simulink model "reaktorChemiczny_20221205_2206"  (R2021b)
settings: Solver=VariableStepAuto  StartTime=0.0  StopTime=10  RelTol=1e-3
model mask{alfa=alfa, ar=ar, cpc=cpc, cpr=cpr, E1=E1, E3=E3, E2=E2, h1=h1, h2=h2, h3=h3, k01=k01, k02=k02, k03=k03, mc=mc, pr=pr, qr=qr, tri=tri, vr=vr}
model workspace (MAT data in the model file):
  E1 = 9800
  E2 = 9800
  E3 = 8600
  Sig = Simulink.Signal
  Sig.DataType = 'auto'
  Sig.Dimensions = -1
  Sig.DimensionsMode = 'auto'
  Sig.Complexity = 'auto'
  Sig.SampleTime = -1
  Sig.SamplingMode = 'auto'
  Sig1 = Simulink.Signal
  Sig1.DataType = 'auto'
  Sig1.Dimensions = -1
  Sig1.DimensionsMode = 'auto'
  Sig1.Complexity = 'auto'
  Sig1.SampleTime = -1
  Sig1.SamplingMode = 'auto'
  alfa = 300
  ar = 0.1
  cpc = 2
  cpr = 3
  h1 = -4200
  h2 = 11000
  h3 = 42000
  k01 = 350000000
  k02 = 350000000
  k03 = 2500000
  mc = 5
  pr = 900
  qr = 0.001
  tri = 393
  vr = 1
settings Model: ParameterArgumentNames=E1,E2,E3,alfa,ar,cpc,cpr,h1,h2,h3,k01,k02,k03,mc,pr,qr,tri,vr  Creator=apple  LastModifiedBy=Black

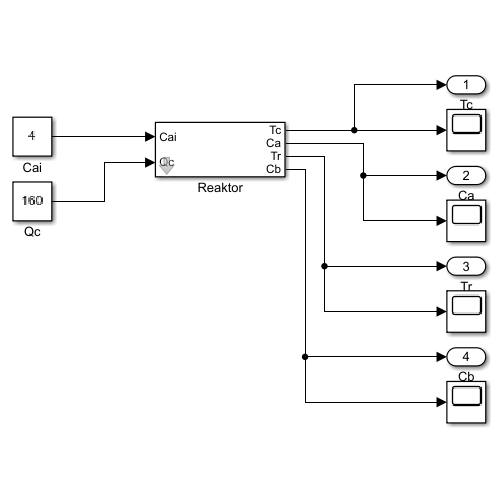
[thumbnail: Simulink's stored preview of the top-level diagram]
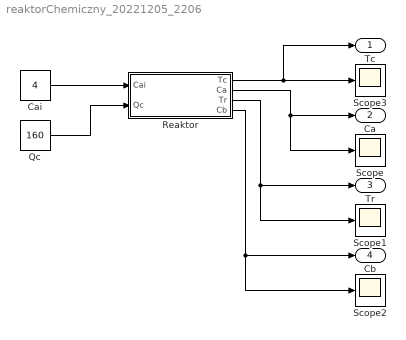
== system reaktorChemiczny_20221205_2206 ==
  Cai : Constant  Value=4
  Qc : Constant  Value=160
  Reaktor : Subsystem  mask{tr0=393, tc0=392, Ca0=5, Cb0=0}
  Scope{,1..3} (4 alike) : Scope
  Tc : Outport
  Ca : Outport  Port=2
  Tr : Outport  Port=3
  Cb : Outport  Port=4
  wires:
  Reaktor/1(Tc) -> Tc/1, Scope3/1
  Reaktor/2(Ca) -> Ca/1, Scope/1
  Reaktor/3(Tr) -> Scope1/1, Tr/1
  Reaktor/4(Cb) -> Scope2/1, Cb/1
  Cai/1 -> Reaktor/1(Cai)
  Qc/1 -> Reaktor/2(Qc)

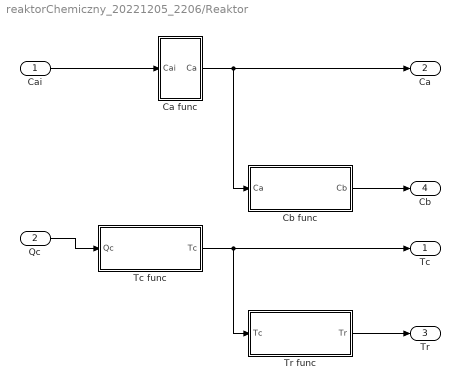
== system reaktorChemiczny_20221205_2206/Reaktor ==
  Cai : Inport  OutMin=0
  Qc : Inport  Port=2  OutMin=0
  Ca func : Subsystem
  Cb func : Subsystem
  Tc func : Subsystem
  Tr func : Subsystem
  Tc : Outport
  Ca : Outport  Port=2
  Tr : Outport  Port=3
  Cb : Outport  Port=4
  wires:
  Tc func/1(Tc) -> Tc/1, Tr func/1(Tc)
  Ca func/1(Ca) -> Cb func/1(Ca), Ca/1
  Cb func/1(Cb) -> Cb/1
  Tr func/1(Tr) -> Tr/1
  Cai/1 -> Ca func/1(Cai)
  Qc/1 -> Tc func/1(Qc)

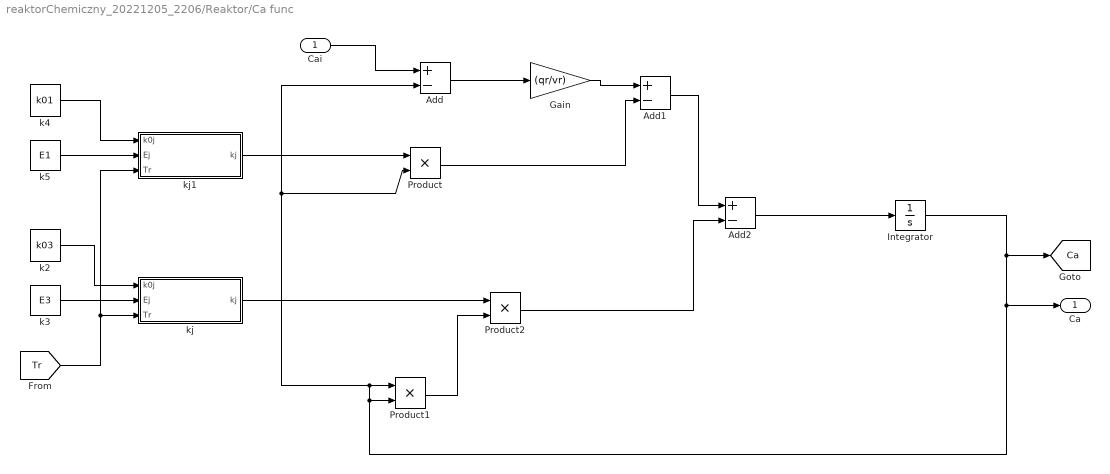
== system reaktorChemiczny_20221205_2206/Reaktor/Ca func ==
  Cai : Inport
  Add : Sum  Inputs=+-
  Add1 : Sum  Inputs=+-
  Add2 : Sum  Inputs=+-
  Gain : Gain  Gain=(qr/vr)
  Integrator : Integrator  InitialCondition=Ca0
  Product : Product
  Product1 : Product
  Product2 : Product
  k2 : Constant  Value=k03
  k3 : Constant  Value=E3
  k4 : Constant  Value=k01
  k5 : Constant  Value=E1
  kj : Subsystem
  kj1 : Subsystem
  Ca : Outport
  tag scope: Ca=global
  wires:
  kj1/1(kj) -> Product/1
  Gain/1 -> Add1/1
  Product1/1 -> Product2/2
  Cai/1 -> Add/1
  Integrator/1 -> [Ca], Ca/1, Product1/1, Add/2, Product/2, Product1/2
  kj/1(kj) -> Product2/1
  Add1/1 -> Add2/1
  Add2/1 -> Integrator/1
  Product2/1 -> Add2/2
  Add/1 -> Gain/1
  Product/1 -> Add1/2
  k3/1 -> kj/2(Ej)
  k2/1 -> kj/1(k0j)
  k5/1 -> kj1/2(Ej)
  k4/1 -> kj1/1(k0j)
  [Tr] -> kj1/3(Tr), kj/3(Tr)

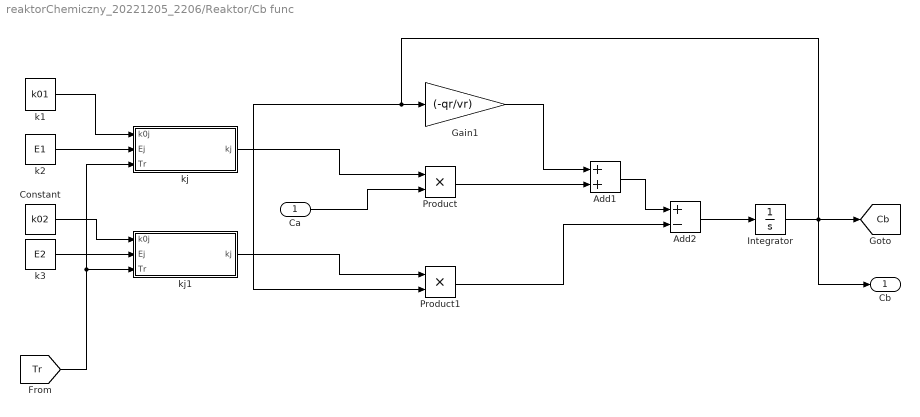
== system reaktorChemiczny_20221205_2206/Reaktor/Cb func ==
  Ca : Inport
  Add1 : Sum
  Add2 : Sum  Inputs=+-
  Constant : Constant  Value=k02
  Gain1 : Gain  Gain=(-qr/vr)
  Integrator : Integrator  InitialCondition=Cb0
  Product : Product
  Product1 : Product
  k1 : Constant  Value=k01
  k2 : Constant  Value=E1
  k3 : Constant  Value=E2
  kj : Subsystem
  kj1 : Subsystem
  Cb : Outport
  tag scope: Cb=global
  wires:
  Add2/1 -> Integrator/1
  Gain1/1 -> Add1/1
  Ca/1 -> Product/2
  Product/1 -> Add1/2
  Integrator/1 -> Product1/2, Gain1/1, [Cb], Cb/1
  Add1/1 -> Add2/1
  Product1/1 -> Add2/2
  k1/1 -> kj/1(k0j)
  Constant/1 -> kj1/1(k0j)
  k2/1 -> kj/2(Ej)
  k3/1 -> kj1/2(Ej)
  [Tr] -> kj1/3(Tr), kj/3(Tr)
  kj1/1(kj) -> Product1/1
  kj/1(kj) -> Product/1

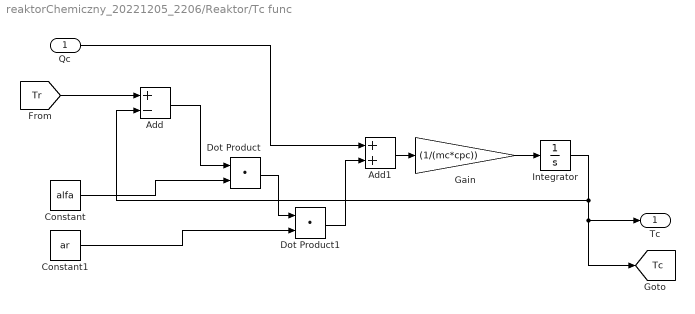
== system reaktorChemiczny_20221205_2206/Reaktor/Tc func ==
  Qc : Inport
  Add : Sum  Inputs=+-
  Add1 : Sum
  Constant : Constant  Value=alfa
  Constant1 : Constant  Value=ar
  Dot Product : DotProduct  InputSameDT=on  OutDataTypeStr=Inherit: Inherit via internal rule
  Dot Product1 : DotProduct  InputSameDT=on  OutDataTypeStr=Inherit: Inherit via internal rule
  Gain : Gain  Gain=(1/(mc*cpc))
  Integrator : Integrator  InitialCondition=tc0
  Tc : Outport
  tag scope: Tc=global
  wires:
  Integrator/1 -> [Tc], Tc/1, Add/2
  Add/1 -> Dot Product/1
  Constant/1 -> Dot Product/2
  Dot Product/1 -> Dot Product1/1
  Constant1/1 -> Dot Product1/2
  Qc/1 -> Add1/1
  Dot Product1/1 -> Add1/2
  Add1/1 -> Gain/1
  Gain/1 -> Integrator/1
  [Tr] -> Add/1

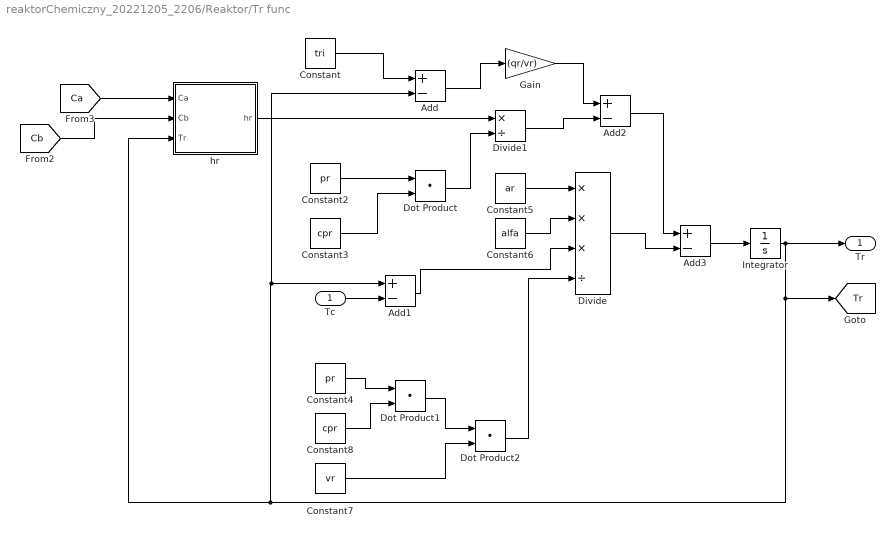
== system reaktorChemiczny_20221205_2206/Reaktor/Tr func ==
  Tc : Inport
  Add{,1..3} (4 alike) : Sum  Inputs=+-
  Constant : Constant  Value=tri
  Constant2 : Constant  Value=pr
  Constant3 : Constant  Value=cpr
  Constant4 : Constant  Value=pr
  Constant5 : Constant  Value=ar
  Constant6 : Constant  Value=alfa
  Constant7 : Constant  Value=vr
  Constant8 : Constant  Value=cpr
  Divide : Product  Inputs=***/
  Divide1 : Product  Inputs=*/
  Dot Product : DotProduct  InputSameDT=on  OutDataTypeStr=Inherit: Inherit via internal rule
  Dot Product1 : DotProduct  InputSameDT=on  OutDataTypeStr=Inherit: Inherit via internal rule
  Dot Product2 : DotProduct  InputSameDT=on  OutDataTypeStr=Inherit: Inherit via internal rule
  Gain : Gain  Gain=(qr/vr)
  Integrator : Integrator  InitialCondition=tr0
  hr : Subsystem
  Tr : Outport
  tag scope: Tr=global
  wires:
  Integrator/1 -> [Tr], Add/2, Add1/1, hr/3(Tr), Tr/1
  Constant/1 -> Add/1
  Constant2/1 -> Dot Product/1
  Constant3/1 -> Dot Product/2
  Dot Product/1 -> Divide1/2
  Divide1/1 -> Add2/2
  Constant5/1 -> Divide/1
  Constant6/1 -> Divide/2
  Add1/1 -> Divide/3
  Constant7/1 -> Dot Product2/2
  Constant4/1 -> Dot Product1/1
  Constant8/1 -> Dot Product1/2
  Dot Product1/1 -> Dot Product2/1
  Dot Product2/1 -> Divide/4
  Tc/1 -> Add1/2
  Divide/1 -> Add3/2
  Add2/1 -> Add3/1
  Add3/1 -> Integrator/1
  Add/1 -> Gain/1
  [Cb] -> hr/2(Cb)
  [Ca] -> hr/1(Ca)
  Gain/1 -> Add2/1
  hr/1(hr) -> Divide1/1

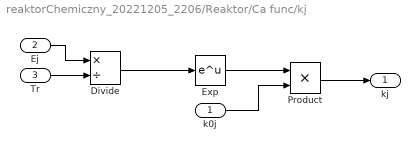
== system reaktorChemiczny_20221205_2206/Reaktor/Ca func/kj ==
  k0j : Inport
  Ej : Inport  Port=2
  Tr : Inport  Port=3
  Divide : Product  Inputs=*/
  Exp : Math  SignedPower=on  SaturateOnIntegerOverflow=on
  Product : Product
  kj : Outport
  wires:
  Product/1 -> kj/1
  Exp/1 -> Product/1
  k0j/1 -> Product/2
  Ej/1 -> Divide/1
  Divide/1 -> Exp/1
  Tr/1 -> Divide/2

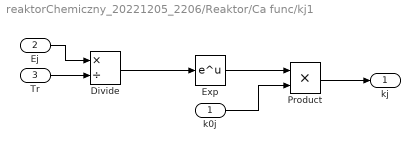
== system reaktorChemiczny_20221205_2206/Reaktor/Ca func/kj1 ==
  k0j : Inport
  Ej : Inport  Port=2
  Tr : Inport  Port=3
  Divide : Product  Inputs=*/
  Exp : Math  SignedPower=on  SaturateOnIntegerOverflow=on
  Product : Product
  kj : Outport
  wires:
  Product/1 -> kj/1
  Exp/1 -> Product/1
  k0j/1 -> Product/2
  Ej/1 -> Divide/1
  Divide/1 -> Exp/1
  Tr/1 -> Divide/2

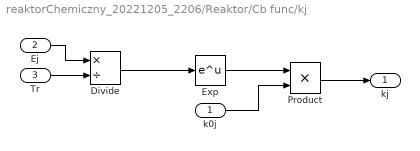
== system reaktorChemiczny_20221205_2206/Reaktor/Cb func/kj ==
  k0j : Inport
  Ej : Inport  Port=2
  Tr : Inport  Port=3
  Divide : Product  Inputs=*/
  Exp : Math  SignedPower=on  SaturateOnIntegerOverflow=on
  Product : Product
  kj : Outport
  wires:
  Product/1 -> kj/1
  Exp/1 -> Product/1
  k0j/1 -> Product/2
  Ej/1 -> Divide/1
  Divide/1 -> Exp/1
  Tr/1 -> Divide/2

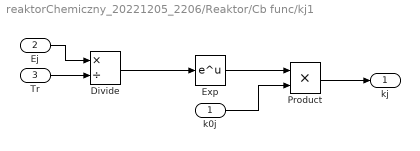
== system reaktorChemiczny_20221205_2206/Reaktor/Cb func/kj1 ==
  k0j : Inport
  Ej : Inport  Port=2
  Tr : Inport  Port=3
  Divide : Product  Inputs=*/
  Exp : Math  SignedPower=on  SaturateOnIntegerOverflow=on
  Product : Product
  kj : Outport
  wires:
  Product/1 -> kj/1
  Exp/1 -> Product/1
  k0j/1 -> Product/2
  Ej/1 -> Divide/1
  Divide/1 -> Exp/1
  Tr/1 -> Divide/2

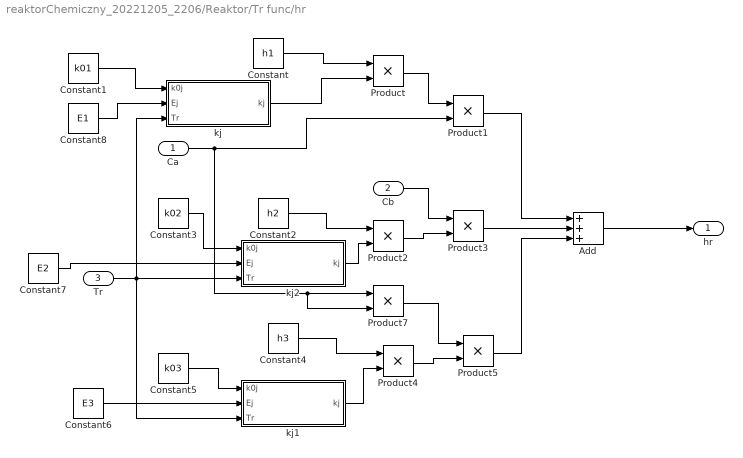
== system reaktorChemiczny_20221205_2206/Reaktor/Tr func/hr ==
  Ca : Inport
  Cb : Inport  Port=2
  Tr : Inport  Port=3
  Add : Sum  Inputs=+++
  Constant : Constant  Value=h1
  Constant1 : Constant  Value=k01
  Constant2 : Constant  Value=h2
  Constant3 : Constant  Value=k02
  Constant4 : Constant  Value=h3
  Constant5 : Constant  Value=k03
  Constant6 : Constant  Value=E3
  Constant7 : Constant  Value=E2
  Constant8 : Constant  Value=E1
  Product{,1..5,7} (7 alike) : Product
  kj : Subsystem
  kj1 : Subsystem
  kj2 : Subsystem
  hr : Outport
  wires:
  Constant/1 -> Product/1
  Product/1 -> Product1/1
  Ca/1 -> Product1/2, Product7/2, Product7/1
  Constant2/1 -> Product2/1
  Product2/1 -> Product3/2
  Cb/1 -> Product3/1
  Product4/1 -> Product5/2
  Constant4/1 -> Product4/1
  Product7/1 -> Product5/1
  Product5/1 -> Add/3
  Product3/1 -> Add/2
  Product1/1 -> Add/1
  Add/1 -> hr/1
  kj/1(kj) -> Product/2
  Constant1/1 -> kj/1(k0j)
  kj1/1(kj) -> Product4/2
  Constant5/1 -> kj1/1(k0j)
  kj2/1(kj) -> Product2/2
  Constant3/1 -> kj2/1(k0j)
  Tr/1 -> kj2/3(Tr), kj/3(Tr), kj1/3(Tr)
  Constant6/1 -> kj1/2(Ej)
  Constant7/1 -> kj2/2(Ej)
  Constant8/1 -> kj/2(Ej)

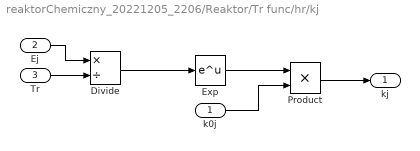
== system reaktorChemiczny_20221205_2206/Reaktor/Tr func/hr/kj ==
  k0j : Inport
  Ej : Inport  Port=2
  Tr : Inport  Port=3
  Divide : Product  Inputs=*/
  Exp : Math  SignedPower=on  SaturateOnIntegerOverflow=on
  Product : Product
  kj : Outport
  wires:
  Product/1 -> kj/1
  Exp/1 -> Product/1
  k0j/1 -> Product/2
  Ej/1 -> Divide/1
  Divide/1 -> Exp/1
  Tr/1 -> Divide/2

== system reaktorChemiczny_20221205_2206/Reaktor/Tr func/hr/kj1 ==
  k0j : Inport
  Ej : Inport  Port=2
  Tr : Inport  Port=3
  Divide : Product  Inputs=*/
  Exp : Math  SignedPower=on  SaturateOnIntegerOverflow=on
  Product : Product
  kj : Outport
  wires:
  Product/1 -> kj/1
  Exp/1 -> Product/1
  k0j/1 -> Product/2
  Ej/1 -> Divide/1
  Divide/1 -> Exp/1
  Tr/1 -> Divide/2

== system reaktorChemiczny_20221205_2206/Reaktor/Tr func/hr/kj2 ==
  k0j : Inport
  Ej : Inport  Port=2
  Tr : Inport  Port=3
  Divide : Product  Inputs=*/
  Exp : Math  SignedPower=on  SaturateOnIntegerOverflow=on
  Product : Product
  kj : Outport
  wires:
  Product/1 -> kj/1
  Exp/1 -> Product/1
  k0j/1 -> Product/2
  Ej/1 -> Divide/1
  Divide/1 -> Exp/1
  Tr/1 -> Divide/2
